simulink model "Series_HEV"  (R2019b)
settings: Solver=VariableStepAuto  StartTime=0.0  StopTime=1061  RelTol=1e-3
undefined symbols (not defined in the file or in its folder): H_u, P_aux, P_CE_cutoff, P_CE_idle, T_CE_cutoff, T_CE_max, theta_CE, V_CE_map, w_CE_idle, w_CE_max, w_CE_upper
libraries: qss_tb_library x8
settings Model: Creator=badk  LastModifiedBy=murugan

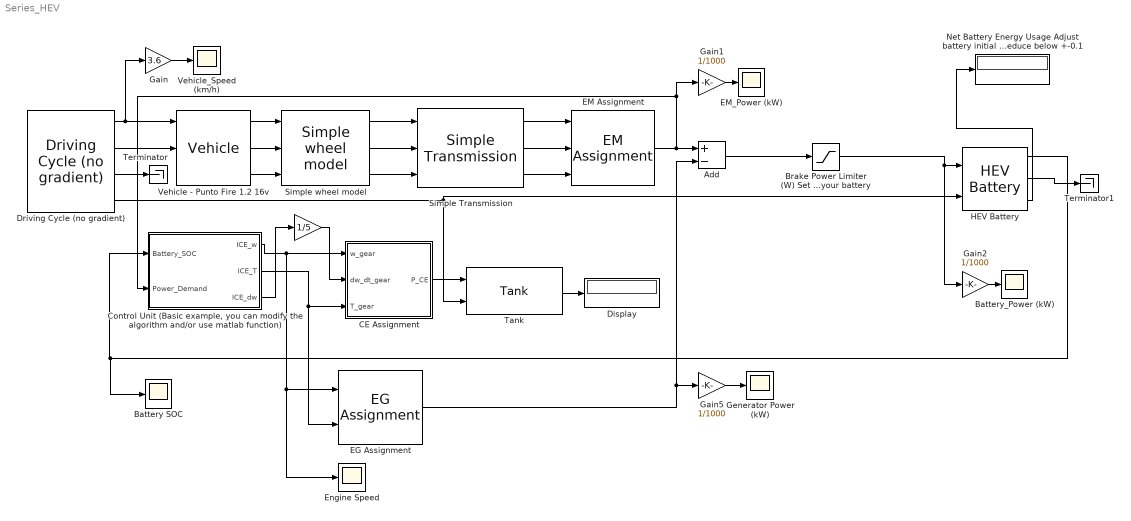
== system Series_HEV ==
  " " : Gain  Gain=1/5
  Add : Sum  Inputs=+-
  Battery SOC : Scope
  Battery_Power (kW) : Scope
  Brake Power Limiter (W) Set a suitable lower value for your battery : Saturate  UpperLimit=500000  LowerLimit=-40000
  CE Assignment : Subsystem  Tag=combustion engine  AncestorBlock=qss_tb_library/Energy Converter/CE Assignment  mask(Combustion Engine (based on consumption map)){engine_type=Gasoline, P_ice=64, ENABLE_FUEL_CUTOFF=on}
      mask prompts: engine_type "Engine type"; P_ice "Power [kW]"; ENABLE_FUEL_CUTOFF "Enable fuel cutoff"
      mask help:
      | This block simulates the behaviour of a combustion engine. The block is based on consumption maps for medium sized passenger cars.
      |
      | NA Gasoline:
      | max power @ 5000 rpm
      | max torque @ 3000 rpm
      |
      | Small Diesel:
      | max power @ 4500 rpm
      | max torque @ 2000 rpm
      |
      | Large Diesel:
      | max power @ 1500 rpm
      | max torque @ 1500 rpm
      |
      |
      | Input:
      | =====
      | 	w_gear	Speed of the fly wheel [rad/s]
      | 	dw_dt_gear	Acceleration of the fly wheel [rad/s^2]
      | 	T_gear	Torque on the fly wheel [Nm]
      |
      | Output:
      | ======
      | 	P_CE	Fuel power consumed by the combustion engine [W]
      mask init:
      | init_AssCE_map;
      mask TypeOptions engine_type: Gasoline | Small Diesel | Large Diesel
  "Control Unit (Basic example, you can modify the algorithm and/or use matlab function)" : Subsystem  Tag=control unit  AncestorBlock=|  mask(Control Unit){}
      | qss_tb_library/Controller/Control Unit
      | (empty template)
      mask help:
      | This block gives the user the opportunity to design his/her own control unit.
      |
      | The user can define the inputs and outputs  by himself/herself.
  Display : Display
  Driving Cycle (no gradient) : qss_tb_library/Driving Cycle/Driving Cycle (no gradient)  Tag=cycle  cyclename1=customcity  stepsize=1  autostop=on
  EG Assignment : qss_tb_library/Energy Converter/EG Assignment  P_eg=35
  EM Assignment : qss_tb_library/Energy Converter/EM Assignment  P_em=46
  EM_Power (kW) : Scope
  Engine Speed : Scope
  Gain : Gain  Gain=3.6
  Gain1 : Gain  Gain=1/1000
  Gain2 : Gain  Gain=1/1000
  Gain5 : Gain  Gain=1/1000
  Generator Power (kW) : Scope
  HEV Battery : qss_tb_library/Energy Buffer/HEV Battery  Tag=battery  cell_series=84  cell_parallel=2  Q_BT_IC_rel=65.5
  Net Battery Energy Usage Adjust battery initial SOC to reduce below +-0.1 : Display
  Simple Transmission : qss_tb_library/Gear System/Simple Transmission  Tag=simple transmission  gear_ratio=4  e_GT=0.98  P_GT0=100  w_wheel_min=1
  Simple wheel model : qss_tb_library/Vehicle/Simple wheel model  Tag=simple transmission  d_wheel=0.5842
  Tank : qss_tb_library/Energy Source/Tank  Tag=tank  fuel=Gasoline  flag_cold_start=on
  Terminator : Terminator
  Terminator1 : Terminator
  Vehicle - Punto Fire 1.2 16v : qss_tb_library/Vehicle/Vehicle  Tag=vehicle  m_f=936+73.5  A_f=(1.48*1.66)  cw=0.31  mu=0.012  k_inertia=4
  Vehicle_Speed (km/h) : Scope
  wires:
  Simple wheel model/3 -> Simple Transmission/3
  Simple Transmission/1 -> EM Assignment/1
  Driving Cycle (no gradient)/2 -> Vehicle - Punto Fire 1.2 16v/2
  Simple Transmission/2 -> EM Assignment/2
  Vehicle - Punto Fire 1.2 16v/1 -> Simple wheel model/1
  Tank/1 -> Display/1
  CE Assignment/1(P_CE) -> Tank/1
  EG Assignment/1 -> Gain5/1, Add/2
  Driving Cycle (no gradient)/4 -> Tank/2, HEV Battery/2
  Gain1/1 -> EM_Power (kW)/1
  Driving Cycle (no gradient)/1 -> Vehicle - Punto Fire 1.2 16v/1, Gain/1
  Add/1 -> Brake Power Limiter (W) Set a suitable lower value for your battery/1
  Brake Power Limiter (W) Set a suitable lower value for your battery/1 -> Gain2/1, HEV Battery/1
  Simple wheel model/1 -> Simple Transmission/1
  Vehicle - Punto Fire 1.2 16v/2 -> Simple wheel model/2
  "Control Unit (Basic example, you can modify the algorithm and/or use matlab function)"/2(ICE_T) -> EG Assignment/2, CE Assignment/3(T_gear)
  Vehicle - Punto Fire 1.2 16v/3 -> Simple wheel model/3
  HEV Battery/3 -> Net Battery Energy Usage Adjust battery initial SOC to reduce below +-0.1/1
  EM Assignment/1 -> Gain1/1, "Control Unit (Basic example, you can modify the algorithm and/or use matlab function)"/2(Power_Demand), Add/1
  "Control Unit (Basic example, you can modify the algorithm and/or use matlab function)"/1(ICE_w) -> Engine Speed/1, EG Assignment/1, CE Assignment/1(w_gear)
  " "/1 -> CE Assignment/2(dw_dt_gear)
  HEV Battery/1 -> "Control Unit (Basic example, you can modify the algorithm and/or use matlab function)"/1(Battery_SOC), Battery SOC/1
  Gain5/1 -> Generator Power (kW)/1
  Gain/1 -> Vehicle_Speed (km/h)/1
  Simple wheel model/2 -> Simple Transmission/2
  Simple Transmission/3 -> EM Assignment/3
  Gain2/1 -> Battery_Power (kW)/1
  "Control Unit (Basic example, you can modify the algorithm and/or use matlab function)"/3("ICE_dw ") -> " "/1
  HEV Battery/2 -> Terminator1/1
  Driving Cycle (no gradient)/3 -> Terminator/1

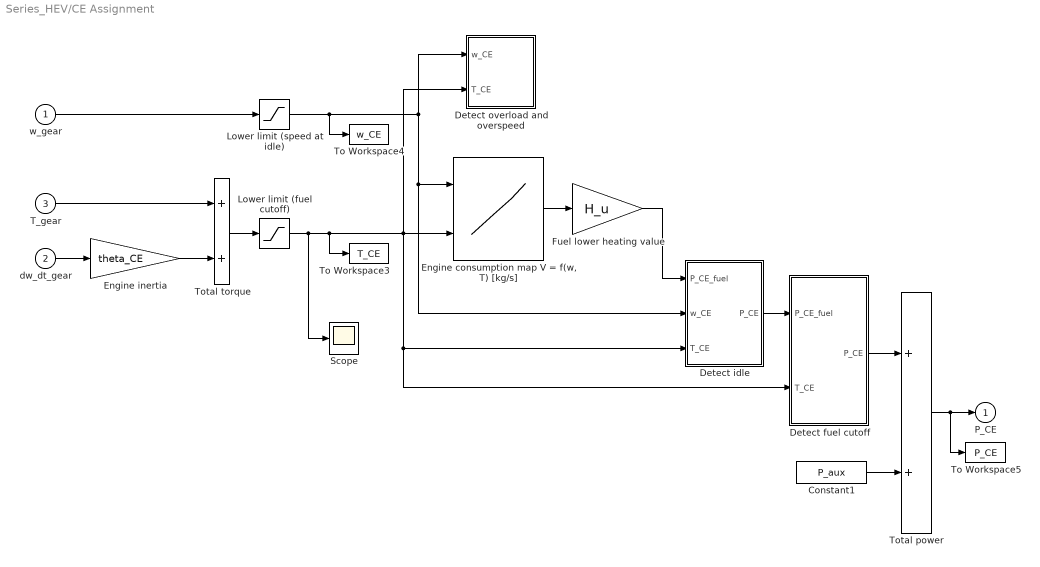
== system Series_HEV/CE Assignment ==
  w_gear : Inport
  dw_dt_gear : Inport  Port=2
  T_gear : Inport  Port=3
  Constant1 : Constant  Value=P_aux
  Detect fuel cutoff : Subsystem
  Detect idle : Subsystem
  Detect overload and overspeed : Subsystem
  "Engine consumption map V = f(w, T) [kg/s]" : Lookup2D  RowIndex=w_CE_row  ColumnIndex=T_CE_col  Table=V_CE_map
  Engine inertia : Gain  Gain=theta_CE  SaturateOnIntegerOverflow=on  OutDataTypeStr=Inherit: Same as input  ParamDataTypeStr=Inherit: Same as input
  Fuel lower heating value : Gain  Gain=H_u  SaturateOnIntegerOverflow=on  OutDataTypeStr=Inherit: Same as input  ParamDataTypeStr=Inherit: Same as input
  Lower limit (fuel cutoff) : Saturate  UpperLimit=inf  LowerLimit=T_CE_cutoff
  Lower limit (speed at idle) : Saturate  UpperLimit=inf  LowerLimit=w_CE_idle
  Scope : Scope
  To Workspace3 : ToWorkspace  VariableName=T_CE  SampleTime=-1
  To Workspace4 : ToWorkspace  VariableName=w_CE  SampleTime=-1
  To Workspace5 : ToWorkspace  VariableName=P_CE  SampleTime=-1
  Total power : Sum  SaturateOnIntegerOverflow=on  InputSameDT=on  OutDataTypeStr=Inherit: Same as first input
  Total torque : Sum  SaturateOnIntegerOverflow=on  InputSameDT=on  OutDataTypeStr=Inherit: Same as first input
  P_CE : Outport  InitialOutput=0
  wires:
  T_gear/1 -> Total torque/1
  dw_dt_gear/1 -> Engine inertia/1
  Total torque/1 -> Lower limit (fuel cutoff)/1
  Engine inertia/1 -> Total torque/2
  Lower limit (speed at idle)/1 -> Detect overload and overspeed/1(w_CE), Detect idle/2(w_CE), "Engine consumption map V = f(w, T) [kg/s]"/1, To Workspace4/1
  w_gear/1 -> Lower limit (speed at idle)/1
  Fuel lower heating value/1 -> Detect idle/1(P_CE_fuel)
  Detect idle/1(P_CE) -> Detect fuel cutoff/1(P_CE_fuel)
  "Engine consumption map V = f(w, T) [kg/s]"/1 -> Fuel lower heating value/1
  Detect fuel cutoff/1(P_CE) -> Total power/1
  Total power/1 -> P_CE/1, To Workspace5/1
  Constant1/1 -> Total power/2
  Lower limit (fuel cutoff)/1 -> Scope/1, Detect overload and overspeed/2(T_CE), "Engine consumption map V = f(w, T) [kg/s]"/2, Detect idle/3(T_CE), Detect fuel cutoff/2(T_CE), To Workspace3/1

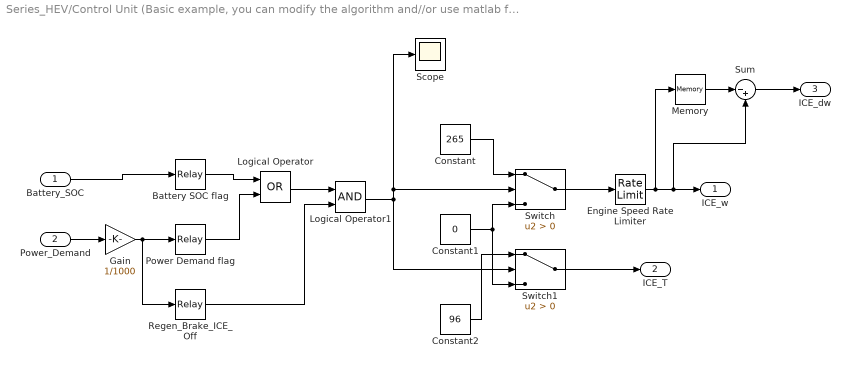
== system Series_HEV/Control Unit (Basic example, you can modify the algorithm and//or use matlab function) ==
  Battery_SOC : Inport
  Power_Demand : Inport  Port=2
  Battery SOC flag : Relay  OnSwitchValue=0.669  OffSwitchValue=0.639  OnOutputValue=0  OffOutputValue=1
  Constant : Constant  Value=265
  Constant1 : Constant  Value=0
  Constant2 : Constant  Value=96
  Engine Speed Rate Limiter : RateLimiter  RisingSlewLimit=150  FallingSlewLimit=-150  SampleTimeMode=inherited
  Gain : Gain  Gain=1/1000
  Logical Operator : Logic  Operator=OR  AllPortsSameDT=off  OutDataTypeStr=boolean
  Logical Operator1 : Logic  AllPortsSameDT=off  OutDataTypeStr=boolean
  Memory : Memory
  Power Demand flag : Relay  OnSwitchValue=20  OffSwitchValue=10
  "Regen_Brake_ICE_Off " : Relay  OnSwitchValue=0  OffSwitchValue=-5
  Scope : Scope
  Sum : Sum  Inputs=|-+
  Switch : Switch  Criteria=u2 > Threshold
  Switch1 : Switch  Criteria=u2 > Threshold
  ICE_w : Outport  InitialOutput=0
  ICE_T : Outport  Port=2  InitialOutput=0
  "ICE_dw " : Outport  Port=3  InitialOutput=0
  wires:
  Battery_SOC/1 -> Battery SOC flag/1
  Battery SOC flag/1 -> Logical Operator/1
  Power Demand flag/1 -> Logical Operator/2
  Logical Operator1/1 -> Scope/1, Switch/2, Switch1/2
  Constant/1 -> Switch/1
  Constant1/1 -> Switch1/3, Switch/3
  Switch1/1 -> ICE_T/1
  Constant2/1 -> Switch1/1
  Power_Demand/1 -> Gain/1
  Gain/1 -> "Regen_Brake_ICE_Off "/1, Power Demand flag/1
  Logical Operator/1 -> Logical Operator1/1
  "Regen_Brake_ICE_Off "/1 -> Logical Operator1/2
  Switch/1 -> Engine Speed Rate Limiter/1
  Engine Speed Rate Limiter/1 -> Memory/1, Sum/2, ICE_w/1
  Memory/1 -> Sum/1
  Sum/1 -> "ICE_dw "/1

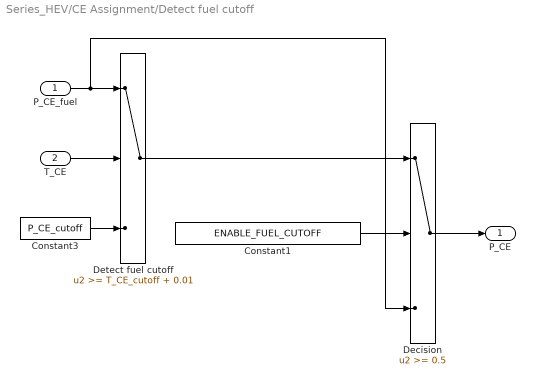
== system Series_HEV/CE Assignment/Detect fuel cutoff ==
  P_CE_fuel : Inport
  T_CE : Inport  Port=2
  Constant1 : Constant  Value=ENABLE_FUEL_CUTOFF
  Constant3 : Constant  Value=P_CE_cutoff
  Decision : Switch  Threshold=0.5
  Detect fuel cutoff : Switch  Threshold=T_CE_cutoff + 0.01  SaturateOnIntegerOverflow=on  InputSameDT=on
  P_CE : Outport
  wires:
  Constant3/1 -> Detect fuel cutoff/3
  T_CE/1 -> Detect fuel cutoff/2
  P_CE_fuel/1 -> Detect fuel cutoff/1, Decision/3
  Detect fuel cutoff/1 -> Decision/1
  Constant1/1 -> Decision/2
  Decision/1 -> P_CE/1

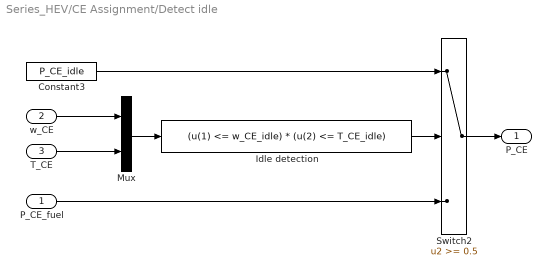
== system Series_HEV/CE Assignment/Detect idle ==
  P_CE_fuel : Inport
  w_CE : Inport  Port=2
  T_CE : Inport  Port=3
  Constant3 : Constant  Value=P_CE_idle
  Idle detection : Fcn  Expr=(u(1) <= w_CE_idle) * (u(2) <= T_CE_idle)
  Mux : Mux  Inputs=2
  Switch2 : Switch  Threshold=0.5  SaturateOnIntegerOverflow=on  InputSameDT=on
  P_CE : Outport  InitialOutput=0
  wires:
  Mux/1 -> Idle detection/1
  T_CE/1 -> Mux/2
  w_CE/1 -> Mux/1
  Idle detection/1 -> Switch2/2
  P_CE_fuel/1 -> Switch2/3
  Switch2/1 -> P_CE/1
  Constant3/1 -> Switch2/1

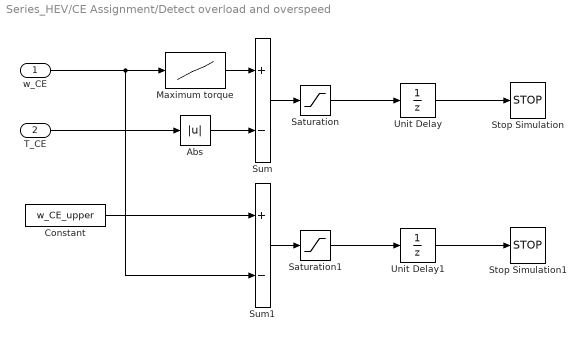
== system Series_HEV/CE Assignment/Detect overload and overspeed ==
  w_CE : Inport
  T_CE : Inport  Port=2
  Abs : Abs  SaturateOnIntegerOverflow=on
  Constant : Constant  Value=w_CE_upper
  Maximum torque : Lookup  InputValues=w_CE_max  Table=T_CE_max  SaturateOnIntegerOverflow=on
  Saturation : Saturate  UpperLimit=0  LowerLimit=-inf
  Saturation1 : Saturate  UpperLimit=0  LowerLimit=-inf
  Stop Simulation : Stop
  Stop Simulation1 : Stop
  Sum : Sum  Inputs=+-  SaturateOnIntegerOverflow=on  InputSameDT=on  OutDataTypeStr=Inherit: Same as first input
  Sum1 : Sum  Inputs=+-  SaturateOnIntegerOverflow=on  InputSameDT=on  OutDataTypeStr=Inherit: Same as first input
  Unit Delay : UnitDelay  SampleTime=-1  HasFrameUpgradeWarning=on
  Unit Delay1 : UnitDelay  SampleTime=-1  HasFrameUpgradeWarning=on
  wires:
  Sum/1 -> Saturation/1
  w_CE/1 -> Maximum torque/1, Sum1/2
  T_CE/1 -> Abs/1
  Maximum torque/1 -> Sum/1
  Abs/1 -> Sum/2
  Saturation/1 -> Unit Delay/1
  Constant/1 -> Sum1/1
  Sum1/1 -> Saturation1/1
  Saturation1/1 -> Unit Delay1/1
  Unit Delay/1 -> Stop Simulation/1
  Unit Delay1/1 -> Stop Simulation1/1
